simulink model "dlbsTestHarnessSigmoid"  (R2025b)
settings: Solver=VariableStepAuto  StartTime=0.0  StopTime=10.0  RelTol=1e-3
undefined symbols (not defined in the file or in its folder): dY, X
libraries: dlbsBlockExtractGradientGF x1, dlbsBlockInsertGradientGF x1, dlbsBlockSigmoid x1
settings Model: Creator=lt6037  LastModifiedBy=lt6037

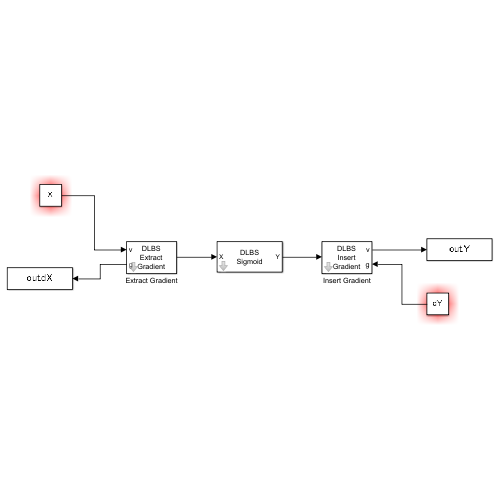
[thumbnail: Simulink's stored preview of the top-level diagram]
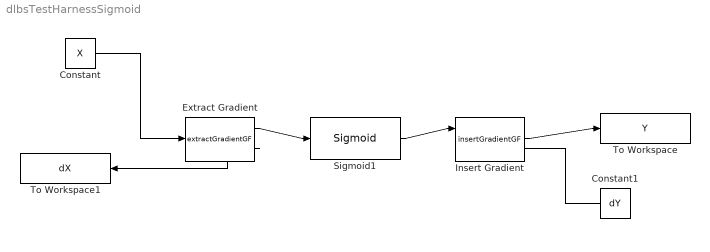
== system dlbsTestHarnessSigmoid ==
  Constant : Constant  Value=X  VectorParams1D=off
  Constant1 : Constant  Value=dY  VectorParams1D=off
  Extract Gradient : dlbsBlockExtractGradientGF/extractGradientGF
  Insert Gradient : dlbsBlockInsertGradientGF/insertGradientGF
  Sigmoid1 : dlbsBlockSigmoid/Sigmoid
  To Workspace : ToWorkspace  VariableName=Y  SaveFormat=Timeseries  SampleTime=-1
      settings: MaxDataPoints=1
  To Workspace1 : ToWorkspace  VariableName=dX  SaveFormat=Timeseries  SampleTime=-1
      settings: MaxDataPoints=1
  wires:
  Extract Gradient/2 -> To Workspace1/1
  Constant1/1 -> Insert Gradient/2
  Constant/1 -> Extract Gradient/1
  Insert Gradient/1 -> To Workspace/1
  Extract Gradient/1 -> Sigmoid1/1
  Sigmoid1/1 -> Insert Gradient/1
